simulink subsystem "Automotive_Suspension_Veh2Tire"  (R2024a)
settings: Solver=VariableStepAuto  StartTime=0.0  StopTime=10.0  RelTol=1e-3
settings Model: Creator=USER  LastModifiedBy=USER

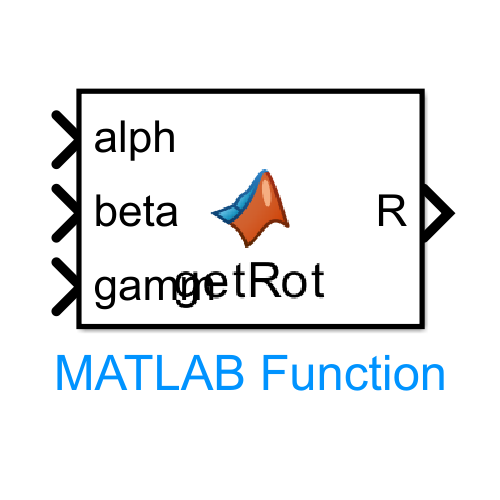
[thumbnail: Simulink's stored preview of the top-level diagram]
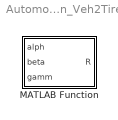
== system Automotive_Suspension_Veh2Tire ==
  MATLAB Function : MATLAB Function  TreatAsAtomicUnit=on

== matlab function Automotive_Suspension_Veh2Tire/MATLAB Function ==
  data: alph input; R output; beta input; gamm input
function R = getRot(alph, beta, gamm)
